simulink model "PMSM20180920"  (Simulink 9.2)
settings: Solver=FixedStepDiscrete  StartTime=0.0  StopTime=Inf  FixedStep=Auto  RelTol=1e-3  EnableMultiTasking=on
undefined symbols (not defined in the file or in its folder): Down, Up
libraries: idelinklib_common x37, c2833xlib x7, c280xlib x6, simulink x3, simulink_extras x2, c2000lib x1
(part 3 of 3)

== system PMSM20180920/Subsystem1/AD/read AD ==
  CH0 : idelinklib_common/Memory Copy  copyFrom=Specified address  copyFromAddressSource=Specify via dialog  copyFromAddress=hex2dec('00200000')  copyFromSrcCode=myVariableSrc  dataTypeFrom=int16  dataDimensionFrom=1  useOffsetFrom=off  offsetFromSrc=Specify via dialog  offsetFrom=0  strideFrom=1  copyTo=Specified source code symbol  copyToAddressSource=Specify via dialog  copyToAddress=hex2dec('00002000')  copyToSrcCode=p1  dataTypeTo=int16  useOffsetTo=off  offsetToSrc=Specify via dialog  offsetTo=0  strideTo=1  sampleTime=inf  useInitValue=off  initValueSrc=Specify constant value  initValue=1  initValueSrcCode=myInitValueVariable  useAsMask=off  maskOperator=bitwise AND  useTermValue=off  termValue=1  isRealtimeEnabled=off  emitCCBeforeWrite=off  CCBeforeWrite=/* Custom Code Before Write*/  emitCCAfterWrite=off  CCAfterWrite=/* Custom Code After Write*/  useDMACopy=off  enableBlockingMode=off
  CH1 : idelinklib_common/Memory Copy  copyFrom=Specified address  copyFromAddressSource=Specify via dialog  copyFromAddress=hex2dec('00200000')  copyFromSrcCode=myVariableSrc  dataTypeFrom=int16  dataDimensionFrom=1  useOffsetFrom=off  offsetFromSrc=Specify via dialog  offsetFrom=0  strideFrom=1  copyTo=Specified source code symbol  copyToAddressSource=Specify via dialog  copyToAddress=hex2dec('00002000')  copyToSrcCode=p2  dataTypeTo=int16  useOffsetTo=off  offsetToSrc=Specify via dialog  offsetTo=0  strideTo=1  sampleTime=inf  useInitValue=off  initValueSrc=Specify constant value  initValue=1  initValueSrcCode=myInitValueVariable  useAsMask=off  maskOperator=bitwise AND  useTermValue=off  termValue=1  isRealtimeEnabled=off  emitCCBeforeWrite=off  CCBeforeWrite=/* Custom Code Before Write*/  emitCCAfterWrite=off  CCAfterWrite=/* Custom Code After Write*/  useDMACopy=off  enableBlockingMode=off
  CH2 : idelinklib_common/Memory Copy  copyFrom=Specified address  copyFromAddressSource=Specify via dialog  copyFromAddress=hex2dec('00200000')  copyFromSrcCode=myVariableSrc  dataTypeFrom=int16  dataDimensionFrom=1  useOffsetFrom=off  offsetFromSrc=Specify via dialog  offsetFrom=0  strideFrom=1  copyTo=Specified source code symbol  copyToAddressSource=Specify via dialog  copyToAddress=hex2dec('00002000')  copyToSrcCode=p3  dataTypeTo=int16  useOffsetTo=off  offsetToSrc=Specify via dialog  offsetTo=0  strideTo=1  sampleTime=inf  useInitValue=off  initValueSrc=Specify constant value  initValue=1  initValueSrcCode=myInitValueVariable  useAsMask=off  maskOperator=bitwise AND  useTermValue=off  termValue=1  isRealtimeEnabled=off  emitCCBeforeWrite=off  CCBeforeWrite=/* Custom Code Before Write*/  emitCCAfterWrite=off  CCAfterWrite=/* Custom Code After Write*/  useDMACopy=off  enableBlockingMode=off
  CH3 : idelinklib_common/Memory Copy  copyFrom=Specified address  copyFromAddressSource=Specify via dialog  copyFromAddress=hex2dec('00200000')  copyFromSrcCode=myVariableSrc  dataTypeFrom=int16  dataDimensionFrom=1  useOffsetFrom=off  offsetFromSrc=Specify via dialog  offsetFrom=0  strideFrom=1  copyTo=Specified source code symbol  copyToAddressSource=Specify via dialog  copyToAddress=hex2dec('00002000')  copyToSrcCode=p4  dataTypeTo=int16  useOffsetTo=off  offsetToSrc=Specify via dialog  offsetTo=0  strideTo=1  sampleTime=inf  useInitValue=off  initValueSrc=Specify constant value  initValue=1  initValueSrcCode=myInitValueVariable  useAsMask=off  maskOperator=bitwise AND  useTermValue=off  termValue=1  isRealtimeEnabled=off  emitCCBeforeWrite=off  CCBeforeWrite=/* Custom Code Before Write*/  emitCCAfterWrite=off  CCAfterWrite=/* Custom Code After Write*/  useDMACopy=off  enableBlockingMode=off
  CH4 : idelinklib_common/Memory Copy  copyFrom=Specified address  copyFromAddressSource=Specify via dialog  copyFromAddress=hex2dec('00200000')  copyFromSrcCode=myVariableSrc  dataTypeFrom=int16  dataDimensionFrom=1  useOffsetFrom=off  offsetFromSrc=Specify via dialog  offsetFrom=0  strideFrom=1  copyTo=Specified source code symbol  copyToAddressSource=Specify via dialog  copyToAddress=hex2dec('00002000')  copyToSrcCode=p5  dataTypeTo=int16  useOffsetTo=off  offsetToSrc=Specify via dialog  offsetTo=0  strideTo=1  sampleTime=inf  useInitValue=off  initValueSrc=Specify constant value  initValue=1  initValueSrcCode=myInitValueVariable  useAsMask=off  maskOperator=bitwise AND  useTermValue=off  termValue=1  isRealtimeEnabled=off  emitCCBeforeWrite=off  CCBeforeWrite=/* Custom Code Before Write*/  emitCCAfterWrite=off  CCAfterWrite=/* Custom Code After Write*/  useDMACopy=off  enableBlockingMode=off
  CH5 : idelinklib_common/Memory Copy  copyFrom=Specified address  copyFromAddressSource=Specify via dialog  copyFromAddress=hex2dec('00200000')  copyFromSrcCode=myVariableSrc  dataTypeFrom=int16  dataDimensionFrom=1  useOffsetFrom=off  offsetFromSrc=Specify via dialog  offsetFrom=0  strideFrom=1  copyTo=Specified source code symbol  copyToAddressSource=Specify via dialog  copyToAddress=hex2dec('00002000')  copyToSrcCode=p6  dataTypeTo=int16  useOffsetTo=off  offsetToSrc=Specify via dialog  offsetTo=0  strideTo=1  sampleTime=inf  useInitValue=off  initValueSrc=Specify constant value  initValue=1  initValueSrcCode=myInitValueVariable  useAsMask=off  maskOperator=bitwise AND  useTermValue=off  termValue=1  isRealtimeEnabled=off  emitCCBeforeWrite=off  CCBeforeWrite=/* Custom Code Before Write*/  emitCCAfterWrite=off  CCAfterWrite=/* Custom Code After Write*/  useDMACopy=off  enableBlockingMode=off
  CH6 : idelinklib_common/Memory Copy  copyFrom=Specified address  copyFromAddressSource=Specify via dialog  copyFromAddress=hex2dec('00200000')  copyFromSrcCode=myVariableSrc  dataTypeFrom=int16  dataDimensionFrom=1  useOffsetFrom=off  offsetFromSrc=Specify via dialog  offsetFrom=0  strideFrom=1  copyTo=Specified source code symbol  copyToAddressSource=Specify via dialog  copyToAddress=hex2dec('00002000')  copyToSrcCode=p7  dataTypeTo=int16  useOffsetTo=off  offsetToSrc=Specify via dialog  offsetTo=0  strideTo=1  sampleTime=inf  useInitValue=off  initValueSrc=Specify constant value  initValue=1  initValueSrcCode=myInitValueVariable  useAsMask=off  maskOperator=bitwise AND  useTermValue=off  termValue=1  isRealtimeEnabled=off  emitCCBeforeWrite=off  CCBeforeWrite=/* Custom Code Before Write*/  emitCCAfterWrite=off  CCAfterWrite=/* Custom Code After Write*/  useDMACopy=off  enableBlockingMode=off
  CH7 : idelinklib_common/Memory Copy  copyFrom=Specified address  copyFromAddressSource=Specify via dialog  copyFromAddress=hex2dec('00200000')  copyFromSrcCode=myVariableSrc  dataTypeFrom=int16  dataDimensionFrom=1  useOffsetFrom=off  offsetFromSrc=Specify via dialog  offsetFrom=0  strideFrom=1  copyTo=Specified source code symbol  copyToAddressSource=Specify via dialog  copyToAddress=hex2dec('00002000')  copyToSrcCode=p8  dataTypeTo=int16  useOffsetTo=off  offsetToSrc=Specify via dialog  offsetTo=0  strideTo=1  sampleTime=inf  useInitValue=off  initValueSrc=Specify constant value  initValue=1  initValueSrcCode=myInitValueVariable  useAsMask=off  maskOperator=bitwise AND  useTermValue=off  termValue=1  isRealtimeEnabled=off  emitCCBeforeWrite=off  CCBeforeWrite=/* Custom Code Before Write*/  emitCCAfterWrite=off  CCAfterWrite=/* Custom Code After Write*/  useDMACopy=off  enableBlockingMode=off
  p1 : idelinklib_common/Memory Copy  copyFrom=Specified source code symbol  copyFromAddressSource=Specify via dialog  copyFromAddress=hex2dec('00200000')  copyFromSrcCode=p1  dataTypeFrom=int16  dataDimensionFrom=1  useOffsetFrom=off  offsetFromSrc=Specify via dialog  offsetFrom=0  strideFrom=1  copyTo=Output port  copyToAddressSource=Specify via dialog  copyToAddress=hex2dec('00002000')  copyToSrcCode=p1  dataTypeTo=int16  useOffsetTo=off  offsetToSrc=Specify via dialog  offsetTo=0  strideTo=1  sampleTime=inf  useInitValue=off  initValueSrc=Specify constant value  initValue=1  initValueSrcCode=myInitValueVariable  useAsMask=off  maskOperator=bitwise AND  useTermValue=off  termValue=1  isRealtimeEnabled=off  emitCCBeforeWrite=off  CCBeforeWrite=/* Custom Code Before Write*/  emitCCAfterWrite=off  CCAfterWrite=/* Custom Code After Write*/  useDMACopy=off  enableBlockingMode=off
  p2 : idelinklib_common/Memory Copy  copyFrom=Specified source code symbol  copyFromAddressSource=Specify via dialog  copyFromAddress=hex2dec('00200000')  copyFromSrcCode=p2  dataTypeFrom=int16  dataDimensionFrom=1  useOffsetFrom=off  offsetFromSrc=Specify via dialog  offsetFrom=0  strideFrom=1  copyTo=Output port  copyToAddressSource=Specify via dialog  copyToAddress=hex2dec('00002000')  copyToSrcCode=p1  dataTypeTo=int16  useOffsetTo=off  offsetToSrc=Specify via dialog  offsetTo=0  strideTo=1  sampleTime=inf  useInitValue=off  initValueSrc=Specify constant value  initValue=1  initValueSrcCode=myInitValueVariable  useAsMask=off  maskOperator=bitwise AND  useTermValue=off  termValue=1  isRealtimeEnabled=off  emitCCBeforeWrite=off  CCBeforeWrite=/* Custom Code Before Write*/  emitCCAfterWrite=off  CCAfterWrite=/* Custom Code After Write*/  useDMACopy=off  enableBlockingMode=off
  p3 : idelinklib_common/Memory Copy  copyFrom=Specified source code symbol  copyFromAddressSource=Specify via dialog  copyFromAddress=hex2dec('00200000')  copyFromSrcCode=p3  dataTypeFrom=int16  dataDimensionFrom=1  useOffsetFrom=off  offsetFromSrc=Specify via dialog  offsetFrom=0  strideFrom=1  copyTo=Output port  copyToAddressSource=Specify via dialog  copyToAddress=hex2dec('00002000')  copyToSrcCode=p1  dataTypeTo=int16  useOffsetTo=off  offsetToSrc=Specify via dialog  offsetTo=0  strideTo=1  sampleTime=inf  useInitValue=off  initValueSrc=Specify constant value  initValue=1  initValueSrcCode=myInitValueVariable  useAsMask=off  maskOperator=bitwise AND  useTermValue=off  termValue=1  isRealtimeEnabled=off  emitCCBeforeWrite=off  CCBeforeWrite=/* Custom Code Before Write*/  emitCCAfterWrite=off  CCAfterWrite=/* Custom Code After Write*/  useDMACopy=off  enableBlockingMode=off
  p5 : idelinklib_common/Memory Copy  copyFrom=Specified source code symbol  copyFromAddressSource=Specify via dialog  copyFromAddress=hex2dec('00200000')  copyFromSrcCode=p5  dataTypeFrom=int16  dataDimensionFrom=1  useOffsetFrom=off  offsetFromSrc=Specify via dialog  offsetFrom=0  strideFrom=1  copyTo=Output port  copyToAddressSource=Specify via dialog  copyToAddress=hex2dec('00002000')  copyToSrcCode=p1  dataTypeTo=int16  useOffsetTo=off  offsetToSrc=Specify via dialog  offsetTo=0  strideTo=1  sampleTime=inf  useInitValue=off  initValueSrc=Specify constant value  initValue=1  initValueSrcCode=myInitValueVariable  useAsMask=off  maskOperator=bitwise AND  useTermValue=off  termValue=1  isRealtimeEnabled=off  emitCCBeforeWrite=off  CCBeforeWrite=/* Custom Code Before Write*/  emitCCAfterWrite=off  CCAfterWrite=/* Custom Code After Write*/  useDMACopy=off  enableBlockingMode=off
  p6 : idelinklib_common/Memory Copy  copyFrom=Specified source code symbol  copyFromAddressSource=Specify via dialog  copyFromAddress=hex2dec('00200000')  copyFromSrcCode=p6  dataTypeFrom=int16  dataDimensionFrom=1  useOffsetFrom=off  offsetFromSrc=Specify via dialog  offsetFrom=0  strideFrom=1  copyTo=Output port  copyToAddressSource=Specify via dialog  copyToAddress=hex2dec('00002000')  copyToSrcCode=p1  dataTypeTo=int16  useOffsetTo=off  offsetToSrc=Specify via dialog  offsetTo=0  strideTo=1  sampleTime=inf  useInitValue=off  initValueSrc=Specify constant value  initValue=1  initValueSrcCode=myInitValueVariable  useAsMask=off  maskOperator=bitwise AND  useTermValue=off  termValue=1  isRealtimeEnabled=off  emitCCBeforeWrite=off  CCBeforeWrite=/* Custom Code Before Write*/  emitCCAfterWrite=off  CCAfterWrite=/* Custom Code After Write*/  useDMACopy=off  enableBlockingMode=off
  p7 : idelinklib_common/Memory Copy  copyFrom=Specified source code symbol  copyFromAddressSource=Specify via dialog  copyFromAddress=hex2dec('00200000')  copyFromSrcCode=p7  dataTypeFrom=int16  dataDimensionFrom=1  useOffsetFrom=off  offsetFromSrc=Specify via dialog  offsetFrom=0  strideFrom=1  copyTo=Output port  copyToAddressSource=Specify via dialog  copyToAddress=hex2dec('00002000')  copyToSrcCode=p1  dataTypeTo=int16  useOffsetTo=off  offsetToSrc=Specify via dialog  offsetTo=0  strideTo=1  sampleTime=inf  useInitValue=off  initValueSrc=Specify constant value  initValue=1  initValueSrcCode=myInitValueVariable  useAsMask=off  maskOperator=bitwise AND  useTermValue=off  termValue=1  isRealtimeEnabled=off  emitCCBeforeWrite=off  CCBeforeWrite=/* Custom Code Before Write*/  emitCCAfterWrite=off  CCAfterWrite=/* Custom Code After Write*/  useDMACopy=off  enableBlockingMode=off
  UD : Outport
  UOUT : Outport  Port=2
  UOUT1 : Outport  Port=3
  FREQ : Outport  Port=4
  IA : Outport  Port=5
  IB : Outport  Port=6
  wires:
  p1/1 -> UD/1
  p2/1 -> UOUT/1
  p3/1 -> UOUT1/1
  p5/1 -> FREQ/1
  p6/1 -> IA/1
  p7/1 -> IB/1

== system PMSM20180920/Subsystem1/PI-ID/RC filter8 ==
  x : Inport
  Constant2 : Constant  Value=a  OutDataTypeStr=double
  Constant3 : Constant  Value=1-a  OutDataTypeStr=double
  Divide : Product
  Divide1 : Product
  Sum2 : Sum
  Unit Delay2 : UnitDelay  SampleTime=-1
  y : Outport
  wires:
  Unit Delay2/1 -> Divide1/2
  Sum2/1 -> Unit Delay2/1, y/1
  Divide1/1 -> Sum2/2
  Divide/1 -> Sum2/1
  Constant3/1 -> Divide1/1
  Constant2/1 -> Divide/2
  x/1 -> Divide/1

== system PMSM20180920/Subsystem1/PI-ID5/RC filter8 ==
  x : Inport
  Constant2 : Constant  Value=a  OutDataTypeStr=double
  Constant3 : Constant  Value=1-a  OutDataTypeStr=double
  Divide : Product
  Divide1 : Product
  Sum2 : Sum
  Unit Delay2 : UnitDelay  SampleTime=-1
  y : Outport
  wires:
  Unit Delay2/1 -> Divide1/2
  Sum2/1 -> Unit Delay2/1, y/1
  Divide1/1 -> Sum2/2
  Divide/1 -> Sum2/1
  Constant3/1 -> Divide1/1
  Constant2/1 -> Divide/2
  x/1 -> Divide/1

== system PMSM20180920/Subsystem1/PI-ID7/RC filter8 ==
  x : Inport
  Constant2 : Constant  Value=a  OutDataTypeStr=double
  Constant3 : Constant  Value=1-a  OutDataTypeStr=double
  Divide : Product
  Divide1 : Product
  Sum2 : Sum
  Unit Delay2 : UnitDelay  SampleTime=-1
  y : Outport
  wires:
  Unit Delay2/1 -> Divide1/2
  Sum2/1 -> Unit Delay2/1, y/1
  Divide1/1 -> Sum2/2
  Divide/1 -> Sum2/1
  Constant3/1 -> Divide1/1
  Constant2/1 -> Divide/2
  x/1 -> Divide/1

== system PMSM20180920/Subsystem1/PI-IQ/RC filter8 ==
  x : Inport
  Constant2 : Constant  Value=a  OutDataTypeStr=double
  Constant3 : Constant  Value=1-a  OutDataTypeStr=double
  Divide : Product
  Divide1 : Product
  Sum2 : Sum
  Unit Delay2 : UnitDelay  SampleTime=-1
  y : Outport
  wires:
  x/1 -> Divide/1
  Constant2/1 -> Divide/2
  Constant3/1 -> Divide1/1
  Divide/1 -> Sum2/1
  Divide1/1 -> Sum2/2
  Sum2/1 -> y/1, Unit Delay2/1
  Unit Delay2/1 -> Divide1/2

== system PMSM20180920/Subsystem1/PI-IQ5/RC filter8 ==
  x : Inport
  Constant2 : Constant  Value=a  OutDataTypeStr=double
  Constant3 : Constant  Value=1-a  OutDataTypeStr=double
  Divide : Product
  Divide1 : Product
  Sum2 : Sum
  Unit Delay2 : UnitDelay  SampleTime=-1
  y : Outport
  wires:
  x/1 -> Divide/1
  Constant2/1 -> Divide/2
  Constant3/1 -> Divide1/1
  Divide/1 -> Sum2/1
  Divide1/1 -> Sum2/2
  Sum2/1 -> y/1, Unit Delay2/1
  Unit Delay2/1 -> Divide1/2

== system PMSM20180920/Subsystem1/PI-IQ7/RC filter8 ==
  x : Inport
  Constant2 : Constant  Value=a  OutDataTypeStr=double
  Constant3 : Constant  Value=1-a  OutDataTypeStr=double
  Divide : Product
  Divide1 : Product
  Sum2 : Sum
  Unit Delay2 : UnitDelay  SampleTime=-1
  y : Outport
  wires:
  x/1 -> Divide/1
  Constant2/1 -> Divide/2
  Constant3/1 -> Divide1/1
  Divide/1 -> Sum2/1
  Divide1/1 -> Sum2/2
  Sum2/1 -> y/1, Unit Delay2/1
  Unit Delay2/1 -> Divide1/2

== system PMSM20180920/Subsystem1/PI-Nr/RC filter8 ==
  x : Inport
  Constant2 : Constant  Value=a  OutDataTypeStr=double
  Constant3 : Constant  Value=1-a  OutDataTypeStr=double
  Divide : Product
  Divide1 : Product
  Sum2 : Sum
  Unit Delay2 : UnitDelay  SampleTime=-1
  y : Outport
  wires:
  Unit Delay2/1 -> Divide1/2
  Sum2/1 -> Unit Delay2/1, y/1
  Divide1/1 -> Sum2/2
  Divide/1 -> Sum2/1
  Constant3/1 -> Divide1/1
  Constant2/1 -> Divide/2
  x/1 -> Divide/1

== system PMSM20180920/Subsystem1/SPWM/Clarke1 ==
  In1 : Inport
  In2 : Inport  Port=2
  Constant58 : Constant  Value=3  OutDataTypeStr=double
  Divide : Product  Inputs=*/
  Gain : Gain  Gain=2
  Gain1 : Gain
  Gain2 : Gain
  Sqrt : Sqrt  SaturateOnIntegerOverflow=on
  Sum : Sum
  alpha : Outport
  beta : Outport  Port=2
  wires:
  Divide/1 -> Gain2/1
  Sqrt/1 -> Divide/2
  Constant58/1 -> Sqrt/1
  Sum/1 -> Divide/1
  Gain/1 -> Sum/2
  In1/1 -> Sum/1, Gain1/1
  In2/1 -> Gain/1
  Gain1/1 -> alpha/1
  Gain2/1 -> beta/1

== system PMSM20180920/Subsystem1/abc/dq current/Clarke1 ==
  In1 : Inport
  In2 : Inport  Port=2
  Constant58 : Constant  Value=3  OutDataTypeStr=double
  Divide : Product  Inputs=*/
  Gain : Gain  Gain=2
  Sqrt : Sqrt  SaturateOnIntegerOverflow=on
  Sum : Sum
  alpha : Outport
  beta : Outport  Port=2
  wires:
  Divide/1 -> beta/1
  Sqrt/1 -> Divide/2
  Constant58/1 -> Sqrt/1
  Sum/1 -> Divide/1
  Gain/1 -> Sum/2
  In1/1 -> Sum/1, alpha/1
  In2/1 -> Gain/1

== system PMSM20180920/Subsystem1/abc/dq current/Park1 ==
  alpha : Inport
  beta : Inport  Port=2
  theta : Inport  Port=3
  Add4 : Sum
  Add5 : Sum
  Gain1 : Gain  Gain=-1
  Product{,1..3} (4 alike) : Product  RndMeth=Zero
  cos : Trigonometry  Operator=cos
  sin : Trigonometry
  d : Outport
  q : Outport  Port=2
  wires:
  Product3/1 -> Add5/2
  Gain1/1 -> Add5/1
  Product2/1 -> Gain1/1
  Product/1 -> Add4/2
  Product1/1 -> Add4/1
  alpha/1 -> Product1/1, Product2/2
  Add4/1 -> d/1
  theta/1 -> cos/1, sin/1
  Add5/1 -> q/1
  cos/1 -> Product1/2, Product3/1
  beta/1 -> Product/2, Product3/2
  sin/1 -> Product/1, Product2/1

== system PMSM20180920/Subsystem1/angle_evalu/PI-ID3 ==
  err : Inport
  reset : Inport  Port=2
  P : Inport  Port=3
  I : Inport  Port=4
  D : Inport  Port=5
  OV : Inport  Port=6
  Constant1 : Constant  Value=0  OutDataTypeStr=Inherit: Inherit via back propagation
  Constant2 : Constant  Value=25  OutDataTypeStr=Inherit: Inherit via back propagation
  Constant3 : Constant  Value=0  OutDataTypeStr=Inherit: Inherit via back propagation
  Constant5 : Constant  Value=0  OutDataTypeStr=Inherit: Inherit via back propagation
  Logical Operator5 : Logic  AllPortsSameDT=off  OutDataTypeStr=boolean
  Logical Operator6 : Logic  Operator=NOT  AllPortsSameDT=off  OutDataTypeStr=boolean
  Product : Product  RndMeth=Zero
  Product1 : Product  RndMeth=Zero
  Product2 : Product  RndMeth=Zero
  RC filter8 : Subsystem  mask{a=0.4}
      mask prompts: a "Time Constant"
  Saturation : Saturate  UpperLimit=max  LowerLimit=min  LinearizeAsGain=off  ZeroCross=off  OutDataTypeStr=double
  Saturation1 : Saturate  UpperLimit=ermax  LowerLimit=ermin  LinearizeAsGain=off  ZeroCross=off  OutDataTypeStr=double
  Saturation2 : Saturate  UpperLimit=max  LowerLimit=min  LinearizeAsGain=off  ZeroCross=off  OutDataTypeStr=double
  Sum1 : Sum  Inputs=+++
  Sum2 : Sum  Inputs=+-
  Sum4 : Sum
  Switch{1..4} (4 alike) : Switch  Criteria=u2 > Threshold  SaturateOnIntegerOverflow=on  InputSameDT=on
  Unit Delay1 : UnitDelay  SampleTime=-1
  Unit Delay3 : UnitDelay  SampleTime=-1
  out : Outport
  wires:
  Logical Operator6/1 -> Logical Operator5/2
  Logical Operator5/1 -> Switch4/2
  RC filter8/1(y) -> Sum1/3
  Constant3/1 -> Switch3/3
  Switch3/1 -> Switch1/3
  Saturation2/1 -> Switch3/1
  Switch1/1 -> out/1
  OV/1 -> Logical Operator6/1, Switch1/2
  Constant2/1 -> Switch1/1
  Sum1/1 -> Saturation2/1
  Product2/1 -> RC filter8/1(x)
  Unit Delay1/1 -> Sum2/2
  D/1 -> Product2/2
  Sum2/1 -> Product2/1
  Switch4/1 -> Unit Delay3/1
  Unit Delay3/1 -> Sum4/2
  Saturation/1 -> Switch4/1, Sum1/2
  Sum4/1 -> Saturation/1
  Product1/1 -> Sum4/1
  I/1 -> Product1/2
  Product/1 -> Sum1/1
  Saturation1/1 -> Switch2/1
  err/1 -> Saturation1/1
  Constant1/1 -> Switch2/3
  reset/1 -> Logical Operator5/1, Switch3/2, Switch2/2
  Switch2/1 -> Unit Delay1/1, Sum2/1, Product1/1, Product/1
  P/1 -> Product/2
  Constant5/1 -> Switch4/3

== system PMSM20180920/Subsystem1/angle_evalu/RC filter3 ==
  x : Inport
  Constant2 : Constant  Value=a  OutDataTypeStr=double
  Constant3 : Constant  Value=1-a  OutDataTypeStr=double
  Divide : Product
  Divide1 : Product
  Sum2 : Sum
  Unit Delay2 : UnitDelay  SampleTime=-1
  y : Outport
  wires:
  Unit Delay2/1 -> Divide1/2
  Sum2/1 -> Unit Delay2/1, y/1
  Divide1/1 -> Sum2/2
  Divide/1 -> Sum2/1
  Constant3/1 -> Divide1/1
  Constant2/1 -> Divide/2
  x/1 -> Divide/1

== system PMSM20180920/Subsystem1/angle_evalu/angle generation ==
  freq : Inport
  Com : simulink/Logic and Bit Operations/Compare To Constant  relop=>=  const=2*pi  OutDataTypeStr=boolean
  Constant3 : Constant  Value=2*pi  OutDataTypeStr=double
  Rem : Math  Operator=rem  SaturateOnIntegerOverflow=on
  Sum11 : Sum
  Switch2 : Switch  Threshold=1
  Unit Delay1 : UnitDelay  SampleTime=-1
  angle_0 : Outport
  wires:
  Unit Delay1/1 -> Sum11/1
  freq/1 -> Sum11/2
  Sum11/1 -> Com/1, Switch2/3, Rem/1
  Switch2/1 -> angle_0/1, Unit Delay1/1
  Com/1 -> Switch2/2
  Rem/1 -> Switch2/1
  Constant3/1 -> Rem/2

== system PMSM20180920/Subsystem1/conversion/RC filter1 ==
  x : Inport
  Constant2 : Constant  Value=a  OutDataTypeStr=double
  Constant3 : Constant  Value=1-a  OutDataTypeStr=double
  Divide : Product
  Divide1 : Product
  Sum2 : Sum
  Unit Delay2 : UnitDelay  SampleTime=-1
  y : Outport
  wires:
  x/1 -> Divide/1
  Constant2/1 -> Divide/2
  Constant3/1 -> Divide1/1
  Divide/1 -> Sum2/1
  Divide1/1 -> Sum2/2
  Sum2/1 -> y/1, Unit Delay2/1
  Unit Delay2/1 -> Divide1/2

== system PMSM20180920/Subsystem1/conversion/RC filter2 ==
  x : Inport
  Constant2 : Constant  Value=a  OutDataTypeStr=double
  Constant3 : Constant  Value=1-a  OutDataTypeStr=double
  Divide : Product
  Divide1 : Product
  Sum2 : Sum
  Unit Delay2 : UnitDelay  SampleTime=-1
  y : Outport
  wires:
  Unit Delay2/1 -> Divide1/2
  Sum2/1 -> Unit Delay2/1, y/1
  Divide1/1 -> Sum2/2
  Divide/1 -> Sum2/1
  Constant3/1 -> Divide1/1
  Constant2/1 -> Divide/2
  x/1 -> Divide/1

== system PMSM20180920/Subsystem1/conversion/RC filter3 ==
  x : Inport
  Constant2 : Constant  Value=a  OutDataTypeStr=double
  Constant3 : Constant  Value=1-a  OutDataTypeStr=double
  Divide : Product
  Divide1 : Product
  Sum2 : Sum
  Unit Delay2 : UnitDelay  SampleTime=-1
  y : Outport
  wires:
  Unit Delay2/1 -> Divide1/2
  Sum2/1 -> Unit Delay2/1, y/1
  Divide1/1 -> Sum2/2
  Divide/1 -> Sum2/1
  Constant3/1 -> Divide1/1
  Constant2/1 -> Divide/2
  x/1 -> Divide/1

== system PMSM20180920/Subsystem1/conversion/RC filter4 ==
  x : Inport
  Constant2 : Constant  Value=a  OutDataTypeStr=double
  Constant3 : Constant  Value=1-a  OutDataTypeStr=double
  Divide : Product
  Divide1 : Product
  Sum2 : Sum
  Unit Delay2 : UnitDelay  SampleTime=-1
  y : Outport
  wires:
  Unit Delay2/1 -> Divide1/2
  Sum2/1 -> Unit Delay2/1, y/1
  Divide1/1 -> Sum2/2
  Divide/1 -> Sum2/1
  Constant3/1 -> Divide1/1
  Constant2/1 -> Divide/2
  x/1 -> Divide/1

== system PMSM20180920/Subsystem1/w_evalu/RC filter4 ==
  x : Inport
  Constant2 : Constant  Value=a  OutDataTypeStr=double
  Constant3 : Constant  Value=1-a  OutDataTypeStr=double
  Divide : Product
  Divide1 : Product
  Sum2 : Sum
  Unit Delay2 : UnitDelay  SampleTime=-1
  y : Outport
  wires:
  x/1 -> Divide/1
  Constant2/1 -> Divide/2
  Constant3/1 -> Divide1/1
  Divide/1 -> Sum2/1
  Divide1/1 -> Sum2/2
  Sum2/1 -> y/1, Unit Delay2/1
  Unit Delay2/1 -> Divide1/2

== system PMSM20180920/Subsystem1/angle_evalu/PI-ID3/RC filter8 ==
  x : Inport
  Constant2 : Constant  Value=a  OutDataTypeStr=double
  Constant3 : Constant  Value=1-a  OutDataTypeStr=double
  Divide : Product
  Divide1 : Product
  Sum2 : Sum
  Unit Delay2 : UnitDelay  SampleTime=-1
  y : Outport
  wires:
  Unit Delay2/1 -> Divide1/2
  Sum2/1 -> Unit Delay2/1, y/1
  Divide1/1 -> Sum2/2
  Divide/1 -> Sum2/1
  Constant3/1 -> Divide1/1
  Constant2/1 -> Divide/2
  x/1 -> Divide/1
